simulink model "AC_asynchronous_motor"  (R2025b)
settings: Solver=VariableStepAuto  StartTime=0.0  StopTime=15  RelTol=1e-3
undefined symbols (not defined in the file): Lm, Lr, Ls, omega_m_const, omega_s_const, p, Rr, Rs, sigma
libraries: nesl_utility x10, ee_lib x8, fl_lib x6
settings Model: Creator=Администратор  LastModifiedBy=Администратор

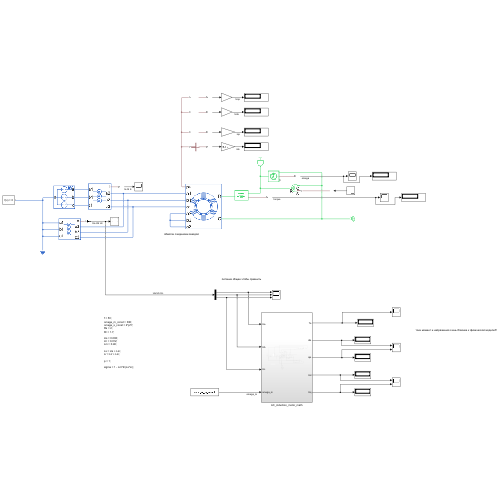
[thumbnail: Simulink's stored preview of the top-level diagram]
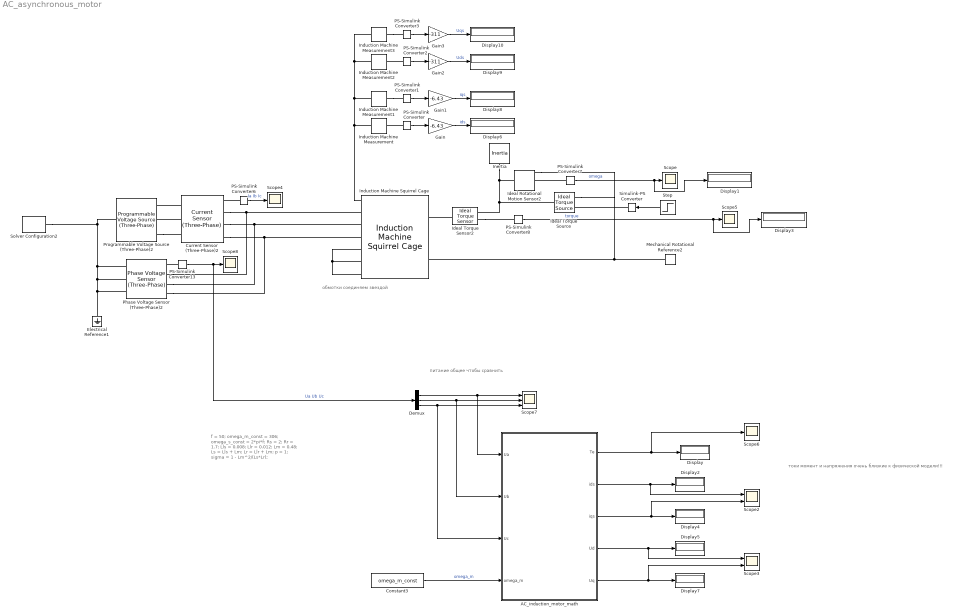
== system AC_asynchronous_motor ==
  note: токи момент и напряжения очень близкие к физической модели!!!
  note: обмотки соединяем звездой
  note: f = 50;
      | omega_m_const = 306;
      | omega_s_const = 2*pi*f;
      | Rs = 2;
      | Rr = 1.7;
      |
      | Lls = 0.008;
      | Llr = 0.012;
      | Lm = 0.48;
      |
      | Ls = Lls + Lm;
      | Lr = Llr + Lm;
      |
      | p = 1;
      |
      | sigma = 1 - Lm^2/(Ls*Lr);
  note: питание общее чтобы сравнить
  AC_induction_motor_math : Subsystem
  Constant3 : Constant  Value=omega_m_const
  Current Sensor (Three-Phase)2 : ee_lib/Sensors & Transducers/Current Sensor (Three-Phase)
      settings: InternalSimscapePortConfiguration="{\"Bottom\":[],\"Left\":[{\"id\":\"a1\",\"label\":\"a1\",\"type\":\"foundation.electrical.electrical\"},{\"id\":\"b1\",\"label\":\"b1\",\"type\":\"foundation.electrical.electrical\"},{\"id\":\"c1\",\"label\":\"c1\",\"type\":\"foundation.electrical.electrical\"}],\"Right\":[{\"id\":\"I_output\",\"label\":\"I\",\"type\":\"output\"},{\"id\":\"a2\",\"label\":\"a2\",\"type\":\"foundation.electrical.electrical\"},{\"id\":\"b2\",\"label\":\"b2\",\"type\":\"foundation.electrical.electrical\"},{\"id\":\"c2\",\"label\":\"c2\",\"type\":\"foundation.electrical.electrical\"}],\"Top\":[]}"
  Demux : Demux  Outputs=3
  Display{,1..10} (11 alike) : Display
  Electrical Reference1 : fl_lib/Electrical/Electrical Elements/Electrical Reference
  Gain : Gain  Gain=-6.43
  Gain1 : Gain  Gain=-6.43
  Gain2 : Gain  Gain=-311
  Gain3 : Gain  Gain=-311
  Ideal Rotational Motion Sensor2 : fl_lib/Mechanical/Mechanical Sensors/Ideal Rotational Motion Sensor  reference=foundation.enum.MeasurementReference.difference  acceleration_port=false  velocity_port=true  position_port=true  wrap_angle=false  offset=0 rad
  Ideal Torque Sensor2 : fl_lib/Mechanical/Mechanical Sensors/Ideal Torque Sensor
  Ideal Torque Source : fl_lib/Mechanical/Mechanical Sources/Ideal Torque Source
  Induction Machine Measurement : ee_lib/Electromechanical/Asynchronous/Induction Machine Measurement  output_idx=6
      settings: InternalSimscapePortConfiguration="{\"Bottom\":[],\"Left\":[{\"id\":\"pu_input\",\"label\":\"pu\",\"type\":\"input\"}],\"Right\":[{\"id\":\"pu_output\",\"label\":\"o\",\"type\":\"output\"}],\"Top\":[]}"
  Induction Machine Measurement1 : ee_lib/Electromechanical/Asynchronous/Induction Machine Measurement  output_idx=7
      settings: InternalSimscapePortConfiguration="{\"Bottom\":[],\"Left\":[{\"id\":\"pu_input\",\"label\":\"pu\",\"type\":\"input\"}],\"Right\":[{\"id\":\"pu_output\",\"label\":\"o\",\"type\":\"output\"}],\"Top\":[]}"
  Induction Machine Measurement2 : ee_lib/Electromechanical/Asynchronous/Induction Machine Measurement  output_idx=3
      settings: InternalSimscapePortConfiguration="{\"Bottom\":[],\"Left\":[{\"id\":\"pu_input\",\"label\":\"pu\",\"type\":\"input\"}],\"Right\":[{\"id\":\"pu_output\",\"label\":\"o\",\"type\":\"output\"}],\"Top\":[]}"
  Induction Machine Measurement3 : ee_lib/Electromechanical/Asynchronous/Induction Machine Measurement  output_idx=4
      settings: InternalSimscapePortConfiguration="{\"Bottom\":[],\"Left\":[{\"id\":\"pu_input\",\"label\":\"pu\",\"type\":\"input\"}],\"Right\":[{\"id\":\"pu_output\",\"label\":\"o\",\"type\":\"output\"}],\"Top\":[]}"
  Induction Machine Squirrel Cage : ee_lib/Electromechanical/Asynchronous/Induction Machine Squirrel Cage  port_option=ee.enum.threePhasePort.expanded  SRated=3000 A*V  VRated=220 V  FRated=50 Hz  nPolePairs=1  param_unit=ee.enum.unit.si  squirrel_cage=ee.enum.squirrelcage.Single  zero_sequence=ee.enum.park.zerosequence.include  initialization_option=ee.enum.asm.initialization.fluxvariables  Rs=2.0 Ohm  Xls=2.513 Ohm  pu_Rs=0.0258  pu_Lls=0.0413  Rrd=1.7 Ohm  Xlrd=3.770 Ohm  pu_Rrd=0.0145  pu_Llrd=0.0424  Rrd1=0.28 Ohm  Xlrd1=0.82 Ohm  Rrd2=0.28 Ohm  Xlrd2=0.82 Ohm  pu_Rrd1=0.0290  pu_Llrd1=0.0848  pu_Rrd2=0.0290  pu_Llrd2=0.0848  Xm=150.80 Ohm  pu_Lm=1.7562  X0=0.4 Ohm  pu_L0=0.0413  saturation_option=ee.enum.saturation.exclude  saturation_i=[0, 4, 9, 18, 25, 34, 50, 68, 95, 120] A  saturation_v=[0, 88, 154, 198, 220, 242, 264, 286, 308, 327] V  pu_saturation_i=[0, .176, .396, .792, 1.1, 1.496, 2.2, 2.992, 4.18, 5.28]  pu_saturation_v=[0, .4, .7, .9, 1, 1.1, 1.2, 1.3, 1.4, 1.4864]  connection_option=ee.enum.Connection.delta  angular_position_specify=off  angular_position_priority=None  angular_position=0 deg  angular_position_nominal_specify=off  angular_position_nominal_value=1  angular_position_nominal_unit=deg  pu_psids_specify=off  pu_psids_priority=None  pu_psids=0  pu_psids_nominal_specify=off  pu_psids_nominal_value=1  pu_psids_nominal_unit=1  pu_psiqs_specify=off  pu_psiqs_priority=None  pu_psiqs=0  pu_psiqs_nominal_specify=off  pu_psiqs_nominal_value=1  pu_psiqs_nominal_unit=1  pu_psi0s_specify=off  pu_psi0s_priority=None  pu_psi0s=0  pu_psi0s_nominal_specify=off  pu_psi0s_nominal_value=1  pu_psi0s_nominal_unit=1  pu_psidr_specify=off  pu_psidr_priority=None  pu_psidr=0  pu_psidr_nominal_specify=off  pu_psidr_nominal_value=1  pu_psidr_nominal_unit=1  pu_psiqr_specify=off  pu_psiqr_priority=None  pu_psiqr=0  pu_psiqr_nominal_specify=off  pu_psiqr_nominal_value=1  pu_psiqr_nominal_unit=1  pu_psidr1_specify=off  pu_psidr1_priority=None  pu_psidr1=0  pu_psidr1_nominal_specify=off  pu_psidr1_nominal_value=1  pu_psidr1_nominal_unit=1  pu_psiqr1_specify=off  pu_psiqr1_priority=None  pu_psiqr1=0  pu_psiqr1_nominal_specify=off  pu_psiqr1_nominal_value=1  pu_psiqr1_nominal_unit=1  pu_psidr2_specify=off  pu_psidr2_priority=None  pu_psidr2=0  pu_psidr2_nominal_specify=off  pu_psidr2_nominal_value=1  pu_psidr2_nominal_unit=1  pu_psiqr2_specify=off  pu_psiqr2_priority=None  pu_psiqr2=0  pu_psiqr2_nominal_specify=off  pu_psiqr2_nominal_value=1  pu_psiqr2_nominal_unit=1  psids_specify=off  psids_priority=None  psids=0 Wb  psids_nominal_specify=off  psids_nominal_value=1  psids_nominal_unit=Wb  psiqs_specify=off  psiqs_priority=None  psiqs=0 Wb  psiqs_nominal_specify=off  psiqs_nominal_value=1  psiqs_nominal_unit=Wb  psi0s_specify=off  psi0s_priority=None  psi0s=0 Wb  psi0s_nominal_specify=off  psi0s_nominal_value=1  psi0s_nominal_unit=Wb  psidr_specify=off  psidr_priority=None  psidr=0 Wb  psidr_nominal_specify=off  psidr_nominal_value=1  psidr_nominal_unit=Wb  psiqr_specify=off  psiqr_priority=None  psiqr=0 Wb  psiqr_nominal_specify=off  psiqr_nominal_value=1  psiqr_nominal_unit=Wb  psidr1_specify=off  psidr1_priority=None  psidr1=0 Wb  psidr1_nominal_specify=off  psidr1_nominal_value=1  psidr1_nominal_unit=Wb  psiqr1_specify=off  psiqr1_priority=None  psiqr1=0 Wb  psiqr1_nominal_specify=off  psiqr1_nominal_value=1  psiqr1_nominal_unit=Wb  psidr2_specify=off  psidr2_priority=None  psidr2=0 Wb  psidr2_nominal_specify=off  psidr2_nominal_value=1  psidr2_nominal_unit=Wb  psiqr2_specify=off  psiqr2_priority=None  psiqr2=0 Wb  psiqr2_nominal_specify=off  psiqr2_nominal_value=1  psiqr2_nominal_unit=Wb  slip_specify=off  slip_priority=None  slip=0  slip_nominal_specify=off  slip_nominal_value=1  slip_nominal_unit=1  real_power_generated_specify=off  real_power_generated_priority=None  real_power_generated=0 W  real_power_generated_nominal_specify=off  real_power_generated_nominal_value=1  real_power_generated_nominal_unit=W  mechanical_power_consumed_specify=off  mechanical_power_consumed_priority=None  mechanical_power_consumed=0 W  mechanical_power_consumed_nominal_specify=off  mechanical_power_consumed_nominal_value=1  mechanical_power_consumed_nominal_unit=W  Tmeas=298.15 K  alpha=3.93e-3 1/K  alpha_cage=4.4e-3 1/K  stator_thermal_mass=100 J/K  rotor_thermal_mass=200 J/K  temperatureA_specify=off  temperatureA_priority=High  temperatureA=25 degC  temperatureA_nominal_specify=off  temperatureA_nominal_value=1  temperatureA_nominal_unit=degC  temperatureB_specify=off  temperatureB_priority=High  temperatureB=25 degC  temperatureB_nominal_specify=off  temperatureB_nominal_value=1  temperatureB_nominal_unit=degC  temperatureC_specify=off  temperatureC_priority=High  temperatureC=25 degC  temperatureC_nominal_specify=off  temperatureC_nominal_value=1  temperatureC_nominal_unit=degC  temperatureR_specify=off  temperatureR_priority=High  temperatureR=25 degC  temperatureR_nominal_specify=off  temperatureR_nominal_value=1  temperatureR_nominal_unit=degC
      settings: InternalSimscapePortConfiguration="{\"Bottom\":[],\"Left\":[{\"id\":\"R\",\"label\":\"R\",\"type\":\"foundation.mechanical.rotational.rotational\"},{\"id\":\"C\",\"label\":\"C\",\"type\":\"foundation.mechanical.rotational.rotational\"}],\"Right\":[{\"id\":\"pu_output\",\"label\":\"pu\",\"type\":\"output\"},{\"id\":\"a1\",\"label\":\"a1\",\"type\":\"foundation.electrical.electrical\"},{\"id\":\"b1\",\"label\":\"b1\",\"type\":\"foundation.electrical.electrical\"},{\"id\":\"c1\",\"label\":\"c1\",\"type\":\"foundation.electrical.electrical\"},{\"id\":\"a2\",\"label\":\"a2\",\"type\":\"foundation.electrical.electrical\"},{\"id\":\"b2\",\"label\":\"b2\",\"type\":\"foundation.electrical.electrical\"},{\"id\":\"c2\",\"label\":\"c2\",\"type\":\"foundation.electrical.electrical\"}],\"Top\":[]}"
  Inertia : fl_lib/Mechanical/Rotational Elements/Inertia  inertia=0.03 kg*m^2  num_ports=foundation.enum.numPorts2.one  w_specify=off  w_priority=High  w=0 rad/s  w_nominal_specify=off  w_nominal_value=1  w_nominal_unit=rad/s  t_specify=off  t_priority=None  t=0 N*m  t_nominal_specify=off  t_nominal_value=1  t_nominal_unit=N*m
  Mechanical Rotational Reference2 : fl_lib/Mechanical/Rotational Elements/Mechanical Rotational Reference
  PS-Simulink Converter{,1..3,6..8,13} (8 alike) : nesl_utility/PS-Simulink Converter  PhysicalDomain=network_engine_domain  SubClassName=ps_output  LeftPortType=input  RightPortType=output  PseudoPeriodic=off  Frequencies=[]  VectorFormat=inherit  Unit=inherit  AffineConversion=off
  Phase Voltage Sensor (Three-Phase)2 : ee_lib/Sensors & Transducers/Phase Voltage Sensor (Three-Phase)
      settings: InternalSimscapePortConfiguration="{\"Bottom\":[],\"Left\":[{\"id\":\"a1\",\"label\":\"a1\",\"type\":\"foundation.electrical.electrical\"},{\"id\":\"b1\",\"label\":\"b1\",\"type\":\"foundation.electrical.electrical\"},{\"id\":\"c1\",\"label\":\"c1\",\"type\":\"foundation.electrical.electrical\"}],\"Right\":[{\"id\":\"V_output\",\"label\":\"V\",\"type\":\"output\"},{\"id\":\"a2\",\"label\":\"a2\",\"type\":\"foundation.electrical.electrical\"},{\"id\":\"b2\",\"label\":\"b2\",\"type\":\"foundation.electrical.electrical\"},{\"id\":\"c2\",\"label\":\"c2\",\"type\":\"foundation.electrical.electrical\"}],\"Top\":[]}"
  Programmable Voltage Source (Three-Phase)2 : ee_lib/Sources/Programmable Voltage Source (Three-Phase)  magnitude_type=ee.enum.timechanging.constant  vline_rms=381 V  magn_ramp=1 V/s  magn_step=1 V  magn_modu_magn=1 V  magn_modu_freq=1 Hz  magn_t1=1 s  magn_t2=2 s  frequency_type=ee.enum.timechanging.constant  freq=50 Hz  freq_ramp=1 Hz/s  freq_step=1 Hz  freq_modu_magn=1 Hz  freq_modu_freq=1 Hz  freq_t1=1 s  freq_t2=2 s  phase_type=ee.enum.timechanging.constant  shift=0 deg  phase_ramp=1 deg/s  phase_step=1 deg  phase_modu_magn=1 deg  phase_modu_freq=1 Hz  phase_t1=1 s  phase_t2=2 s  impedance_option=1  SShortCircuit=1e6 A*V  XR=15  R=0.01 Ohm  L=3.97e-4 H  G_parasitic=1e-6 1/Ohm  harmonic_option=0  harmonic_orders=[5, 7, 11, 13]  harmonic_ratios=[.1, .1, .1, .1]  harmonic_shifts=[0, 0, 0, 0] deg  harmonic_sequences=[1, 1, 1, 1]  harmonic_t1=-inf s  harmonic_t2=inf s  I_specify=off  I_priority=None  I=[0, 0, 0] A  I_nominal_specify=off  I_nominal_value=1  I_nominal_unit=A  V_specify=off  V_priority=None  V=[0, 0, 0] V  V_nominal_specify=off  V_nominal_value=1  V_nominal_unit=V
      settings: InternalSimscapePortConfiguration="{\"Bottom\":[],\"Left\":[{\"id\":\"n\",\"label\":\"n\",\"type\":\"foundation.electrical.electrical\"}],\"Right\":[{\"id\":\"a\",\"label\":\"a\",\"type\":\"foundation.electrical.electrical\"},{\"id\":\"b\",\"label\":\"b\",\"type\":\"foundation.electrical.electrical\"},{\"id\":\"c\",\"label\":\"c\",\"type\":\"foundation.electrical.electrical\"}],\"Top\":[]}"
  Scope{,4..6,8} (5 alike) : Scope
      Scope settings: ActiveDisplayYMinimum=-377.92659102363564  ActiveDisplayYMaximum=481.30829410991862  DataLoggingVariableName=ScopeData4
      Scope4 settings: ActiveDisplayYMinimum=-283.18935621511253  ActiveDisplayYMaximum=90.573418944669029  DataLoggingVariableName=ScopeData3
      Scope5 settings: ActiveDisplayYMinimum=-58.008737485932372  ActiveDisplayYMaximum=49.203178926662162  DataLoggingVariableName=ScopeData5
      Scope6 settings: ActiveDisplayYMinimum=-1484.7128170140834  ActiveDisplayYMaximum=2478.9693200354709  DataLoggingVariableName=ScopeData6
      Scope8 settings: ActiveDisplayYMinimum=-283.18935621511253  ActiveDisplayYMaximum=90.573418944669029  DataLoggingVariableName=ScopeData8
  Scope2 : Scope  NumInputPorts=2
      settings: ActiveDisplayYMinimum=-287.232762518808  ActiveDisplayYMaximum=32.680439627919853
  Scope3 : Scope  NumInputPorts=2
      settings: ActiveDisplayYMinimum=-688.36948573221423  ActiveDisplayYMaximum=823.2908720056123  DataLoggingVariableName=ScopeData2
  Scope7 : Scope  NumInputPorts=3
      settings: ActiveDisplayYMinimum=-101.07546383187821  ActiveDisplayYMaximum=434.78911607405013  DataLoggingVariableName=ScopeData7
  Simulink-PS Converter : nesl_utility/Simulink-PS Converter  PhysicalDomain=network_engine_domain  SubClassName=ps_input  LeftPortType=input  RightPortType=output  PseudoPeriodic=off  Frequencies=[]  NoiseDistribution=none  NoiseParameters=[]  Unit=1  AffineConversion=off  FilteringAndDerivatives=provide  SimscapeFilterOrder=1  InputFilterTimeConstant=0.001  UdotUserProvided=0
  Solver Configuration2 : nesl_utility/Solver Configuration  PhysicalDomain=network_engine_domain  SubClassName=solver  LeftPortType=input  RightPortType=generic  Tones=[]  Harmonics=[]  SimulateNoise=off  Profile=off  UseLocalSampling=off  EnableSwitchedLinearOptims=on  FrequencyDomain=off  UseCCode=off  RelTol=0.001  AbsTol=0.001  MinStep=1e-09  ToWorkspace=off  RevertToSquareIcSolve=off  NumHomotopyIterations=100  PhasorMode=off  PhasorModeNumHarmonics=1  ConsistencySolver=NEWTON_XTOL_AFTER_FTOL  IndexReductionMethod=DerivativeReplacement  DoDC=off  ResidualTolerance=1e-09  ConsistencyTolSource=GLOBAL  ConsistencyAbsTol=0.001  ConsistencyRelTol=0.001  ConsistencyTolFactor=0.001  UseLocalSolver=off  LocalSolverChoice=NE_BACKWARD_EULER_ADVANCER  ResolveIndetEquations=on  FunctionEvalNumThread=1  LocalSolverSampleTime=0.001  DoFixedCost=off  MaxNonlinIter=3  MaxModeIter=2  ComputeImpulses=off  ImpulseIterations=2  LinearAlgebra=auto  LinearAlgebraNumThread=0  EquationFormulation=NE_TIME_EF  DelaysMemoryBudget=1024  AutomaticFiltering=on  FilteringTimeConstant=0.001  PartitionStorageMethod=AS_NEEDED  PartitionMemoryBudget=1024  PartitionMethod=ROBUST  MultibodyUseLocalSolver=off  MultibodyLocalSolverChoice=ODE1  MultibodyLocalSolverSampleTime=0.001
  Step : Step  Time=5  After=-10  SampleTime=0
  wires:
  PS-Simulink Converter6/1 -> Scope4/1  "Ia Ib Ic"
  PS-Simulink Converter7/1 -> Display1/1, Scope/1  "omega"
  PS-Simulink Converter8/1 -> Display3/1, Scope5/1  "torque"
  Step/1 -> Simulink-PS Converter/1
  Demux/2 -> AC_induction_motor_math/2(Ub), Scope7/2
  AC_induction_motor_math/4(Ud) -> Display5/1, Scope3/1
  AC_induction_motor_math/3(iqs) -> Display4/1, Scope2/2
  AC_induction_motor_math/2(ids) -> Display2/1, Scope2/1
  AC_induction_motor_math/5(Uq) -> Scope3/2, Display7/1
  AC_induction_motor_math/1(Te) -> Display/1, Scope6/1
  Demux/3 -> AC_induction_motor_math/3(Uc), Scope7/3
  Constant3/1 -> AC_induction_motor_math/4(omega_m)  "omega_m"
  PS-Simulink Converter13/1 -> Demux/1, Scope8/1  "Ua Ub Uc"
  Demux/1 -> Scope7/1, AC_induction_motor_math/1(Ua)
  PS-Simulink Converter/1 -> Gain/1
  PS-Simulink Converter1/1 -> Gain1/1
  Gain/1 -> Display6/1  "ids"
  Gain1/1 -> Display8/1  "iqs"
  Gain3/1 -> Display10/1  "Uqs"
  Gain2/1 -> Display9/1  "Uds"
  PS-Simulink Converter3/1 -> Gain3/1
  PS-Simulink Converter2/1 -> Gain2/1
  connections:
  PS-Simulink Converter6/LConn1 -- Current Sensor (Three-Phase)2/RConn1
  Current Sensor (Three-Phase)2/LConn1 -- Programmable Voltage Source (Three-Phase)2/RConn1
  Programmable Voltage Source (Three-Phase)2/RConn3 -- Current Sensor (Three-Phase)2/LConn3
  Current Sensor (Three-Phase)2/LConn2 -- Programmable Voltage Source (Three-Phase)2/RConn2
  Induction Machine Squirrel Cage/RConn5 -- Induction Machine Squirrel Cage/RConn6 -- Induction Machine Squirrel Cage/RConn7
  Current Sensor (Three-Phase)2/RConn2 -- Phase Voltage Sensor (Three-Phase)2/RConn2 -- Induction Machine Squirrel Cage/RConn2
  Current Sensor (Three-Phase)2/RConn3 -- Phase Voltage Sensor (Three-Phase)2/RConn3 -- Induction Machine Squirrel Cage/RConn3
  Current Sensor (Three-Phase)2/RConn4 -- Induction Machine Squirrel Cage/RConn4 -- Phase Voltage Sensor (Three-Phase)2/RConn4
  Programmable Voltage Source (Three-Phase)2/LConn1 -- Solver Configuration2/RConn1 -- Phase Voltage Sensor (Three-Phase)2/LConn1 -- Phase Voltage Sensor (Three-Phase)2/LConn2 -- Phase Voltage Sensor (Three-Phase)2/LConn3 -- Electrical Reference1/LConn1
  Ideal Torque Sensor2/LConn1 -- Induction Machine Squirrel Cage/LConn1
  Ideal Rotational Motion Sensor2/LConn1 -- Ideal Torque Sensor2/RConn1 -- Ideal Torque Source/LConn1 -- Inertia/LConn1
  Mechanical Rotational Reference2/LConn1 -- Ideal Torque Source/RConn2 -- Ideal Rotational Motion Sensor2/RConn1 -- Induction Machine Squirrel Cage/LConn2
  PS-Simulink Converter7/LConn1 -- Ideal Rotational Motion Sensor2/RConn2
  Ideal Torque Sensor2/RConn2 -- PS-Simulink Converter8/LConn1
  Simulink-PS Converter/RConn1 -- Ideal Torque Source/RConn1
  Induction Machine Measurement3/LConn1 -- Induction Machine Squirrel Cage/RConn1 -- Induction Machine Measurement/LConn1 -- Induction Machine Measurement1/LConn1 -- Induction Machine Measurement2/LConn1
  PS-Simulink Converter13/LConn1 -- Phase Voltage Sensor (Three-Phase)2/RConn1
  PS-Simulink Converter/LConn1 -- Induction Machine Measurement/RConn1
  Induction Machine Measurement1/RConn1 -- PS-Simulink Converter1/LConn1
  PS-Simulink Converter2/LConn1 -- Induction Machine Measurement2/RConn1
  Induction Machine Measurement3/RConn1 -- PS-Simulink Converter3/LConn1

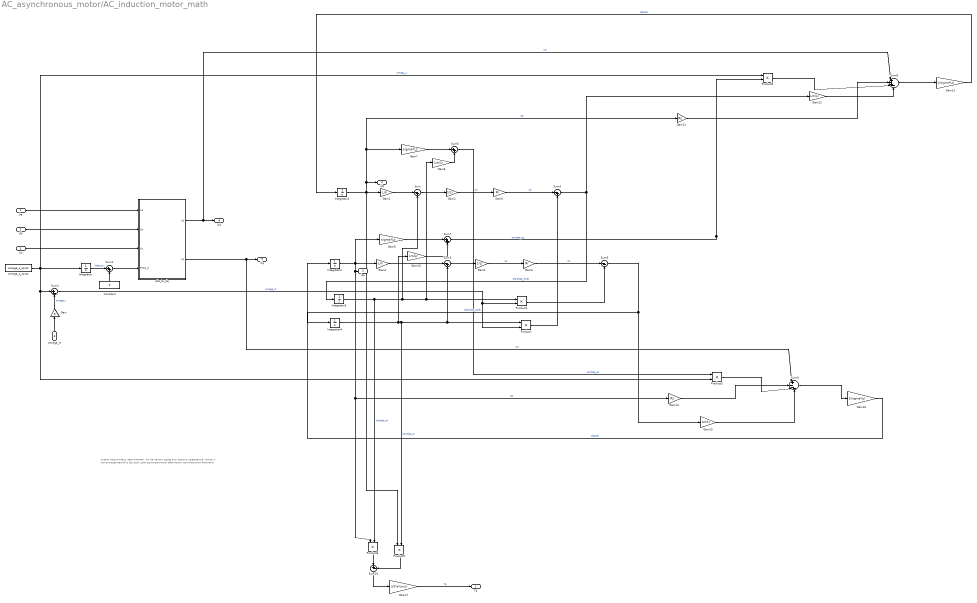
== system AC_asynchronous_motor/AC_induction_motor_math ==
  note: схема получилась запутанная, но на самом деле это просто уравнения токов и потокосцеплений в dq осях для асинхронника обычными логическими блоками
  Ua : Inport
  Ub : Inport  Port=2
  Uc : Inport  Port=3
  omega_m : Inport  Port=4
  Constant : Constant  Value=0
  Gain : Gain  Gain=p
  Gain1 : Gain  Gain=Lm
  Gain{8,10,12,15} (4 alike) : Gain  Gain=Lm/Lr
  Gain11 : Gain  Gain=Rs
  Gain13 : Gain  Gain=1/(sigma*Ls)
  Gain14 : Gain  Gain=Rs
  Gain16 : Gain  Gain=1/(sigma*Ls)
  Gain17 : Gain  Gain=3/2*p*Lm/Lr
  Gain2 : Gain  Gain=1/Lr
  Gain3 : Gain  Gain=Lm
  Gain4 : Gain  Gain=1/Lr
  Gain5 : Gain  Gain=Rr
  Gain6 : Gain  Gain=Rr
  Gain7 : Gain  Gain=sigma*Ls
  Gain9 : Gain  Gain=sigma*Ls
  Integrator{,1..4} (5 alike) : Integrator
  Product{,1..5} (6 alike) : Product
  Sum : Sum  Inputs=|-+
  Sum1 : Sum  Inputs=|++
  Sum10 : Sum  Inputs=|+-
  Sum2 : Sum  Inputs=|+-
  Sum3 : Sum  Inputs=|-+
  Sum4 : Sum  Inputs=|-+
  Sum5 : Sum  Inputs=|--
  Sum6 : Sum  Inputs=|++
  Sum7 : Sum  Inputs=|++
  Sum8 : Sum  Inputs=|+-+-
  Sum9 : Sum  Inputs=|+---
  abc_to_dq : Subsystem
  omega_s_const : Constant  Value=omega_s_const
  Te : Outport
  ids : Outport  Port=2
  iqs : Outport  Port=3
  Ud : Outport  Port=4
  Uq : Outport  Port=5
  wires:
  omega_m/1 -> Gain/1
  Integrator/1 -> Sum1/1  "theta_e"
  Ua/1 -> abc_to_dq/1(Ua)
  Ub/1 -> abc_to_dq/2(Ub)
  Uc/1 -> abc_to_dq/3(Uc)
  abc_to_dq/1(Ud) -> Ud/1, Sum8/1  "Ud"
  abc_to_dq/2(Uq) -> Uq/1, Sum9/1  "Uq"
  Integrator1/1 -> ids/1, Gain7/1, Gain11/1, Product5/1, Gain1/1  "ids"
  Integrator2/1 -> iqs/1, Gain14/1, Product4/1, Gain3/1, Gain9/1  "iqs"
  Sum1/1 -> abc_to_dq/4(theta_e)
  Constant/1 -> Sum1/2
  omega_s_const/1 -> Integrator/1, Product2/1, Sum2/1, Product3/2  "omega_s"
  Gain/1 -> Sum2/2  "omega_r"
  Sum2/1 -> Product/2, Product1/2  "omega_sl"
  Gain16/1 -> Integrator2/1  "diqs/dt"
  Sum4/1 -> Gain12/1, Integrator3/1  "dlambda_dr/dt"
  Integrator3/1 -> Product1/1, Gain8/1, Sum/2, Product4/2  "lambda_dr"
  Sum5/1 -> Gain15/1, Integrator4/1  "dlambda_qr/dt"
  Integrator4/1 -> Product/1, Sum3/2, Product5/2, Gain10/1  "lambda_qr"
  Gain1/1 -> Sum/1
  Sum/1 -> Gain2/1
  Gain2/1 -> Gain5/1  "idr"
  Gain3/1 -> Sum3/1
  Sum3/1 -> Gain4/1
  Gain4/1 -> Gain6/1  "iqr"
  Gain5/1 -> Sum4/1  "idr"
  Product/1 -> Sum4/2
  Product1/1 -> Sum5/2
  Gain6/1 -> Sum5/1  "idr"
  Gain8/1 -> Sum6/2
  Gain7/1 -> Sum6/1
  Sum6/1 -> Product3/1  "lambda_ds"
  Gain9/1 -> Sum7/1
  Gain10/1 -> Sum7/2
  Sum7/1 -> Product2/2  "lambda_qs"
  Gain11/1 -> Sum8/2
  Product2/1 -> Sum8/3
  Gain12/1 -> Sum8/4
  Sum8/1 -> Gain13/1
  Gain13/1 -> Integrator1/1  "dids/dt"
  Gain14/1 -> Sum9/2
  Product3/1 -> Sum9/3
  Gain15/1 -> Sum9/4
  Sum9/1 -> Gain16/1
  Product4/1 -> Sum10/1
  Product5/1 -> Sum10/2
  Sum10/1 -> Gain17/1
  Gain17/1 -> Te/1  "Te"

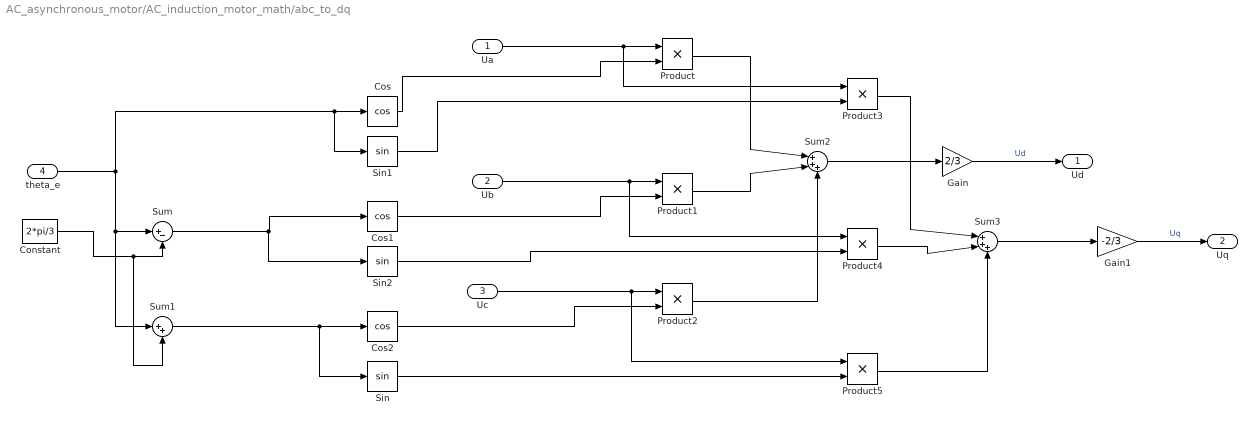
== system AC_asynchronous_motor/AC_induction_motor_math/abc_to_dq ==
  Ua : Inport
  Ub : Inport  Port=2
  Uc : Inport  Port=3
  theta_e : Inport  Port=4
  Constant : Constant  Value=2*pi/3
  Cos : Trigonometry  Operator=cos
  Cos1 : Trigonometry  Operator=cos
  Cos2 : Trigonometry  Operator=cos
  Gain : Gain  Gain=2/3
  Gain1 : Gain  Gain=-2/3
  Product{,1..5} (6 alike) : Product
  Sin : Trigonometry
  Sin1 : Trigonometry
  Sin2 : Trigonometry
  Sum : Sum  Inputs=|+-
  Sum1 : Sum  Inputs=|++
  Sum2 : Sum  Inputs=|+++
  Sum3 : Sum  Inputs=|+++
  Ud : Outport
  Uq : Outport  Port=2
  wires:
  theta_e/1 -> Sum1/1, Sum/1, Sin1/1, Cos/1
  Constant/1 -> Sum1/2, Sum/2
  Cos/1 -> Product/2
  Ua/1 -> Product3/1, Product/1
  Sum/1 -> Sin2/1, Cos1/1
  Ub/1 -> Product4/1, Product1/1
  Sum1/1 -> Sin/1, Cos2/1
  Uc/1 -> Product5/1, Product2/1
  Cos1/1 -> Product1/2
  Cos2/1 -> Product2/2
  Product/1 -> Sum2/1
  Product1/1 -> Sum2/2
  Product2/1 -> Sum2/3
  Sum2/1 -> Gain/1
  Gain/1 -> Ud/1  "Ud"
  Sin1/1 -> Product3/2
  Sin2/1 -> Product4/2
  Sin/1 -> Product5/2
  Product3/1 -> Sum3/1
  Product4/1 -> Sum3/2
  Product5/1 -> Sum3/3
  Sum3/1 -> Gain1/1
  Gain1/1 -> Uq/1  "Uq"
